simulink model "PROJETOFINALmotor"  (R2021a)
settings: Solver=VariableStepAuto  StartTime=0  StopTime=144  FixedStep=0.1  RelTol=1e-3
model workspace (MAT data in the model file):
  variavelteste = 0
libraries: autolibsharedmappedengines x2, spsACVoltageSourceLib x1, spsCurrentMeasurementLib x1, spsSeriesRLCBranchLib x1, spspowerguiLib x1
(part 2 of 4)

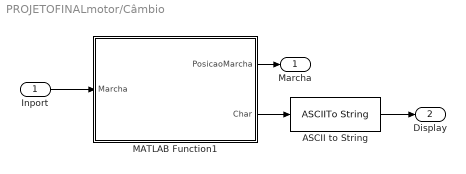
== system PROJETOFINALmotor/Câmbio ==
  Inport : Inport
  ASCII to String : ASCIIToString
  MATLAB Function1 : MATLAB Function  TreatAsAtomicUnit=on
  Marcha : Outport
  Display : Outport  Port=2
  wires:
  MATLAB Function1/1(PosicaoMarcha) -> Marcha/1
  MATLAB Function1/2(Char) -> ASCII to String/1
  ASCII to String/1 -> Display/1
  Inport/1 -> MATLAB Function1/1(Marcha)

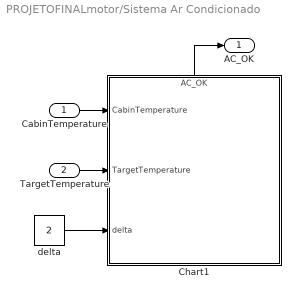
== system PROJETOFINALmotor/Sistema Ar Condicionado ==
  CabinTemperature : Inport
  TargetTemperature : Inport  Port=2
  Chart1 : Stateflow chart  TreatAsAtomicUnit=on
      settings: PortSchema="{\"entries\":[{\"content\":{\"sides\":[{\"content\":{\"connectorIds\":[\"In1\",\"In2\",\"In3\"]},\"type\":\"ConnectorPlacement.EquallySpacedRectSide\",\"uuid\":\"3dcc586e-91d0-4cd1-aed7-6dda3adf5149\"},{\"content\":{\"side\":\"RIGHT\"},\"type\":\"ConnectorPlacement.EquallySpacedRectSide\",\"uuid\":\"6a827bb4-538e-49ed-9fcc-bcf1675a0976\"},{\"content\":{\"connectorIds\":[\"Out1\"],\"side\":\"TOP\"},\"type\":\"ConnectorPlacement.EquallySpacedRectSide\",\"uuid\":\"8af03e4c-b384-4eb2-b8cc-d6be61dc8da4\"}]},\"type\":\"ConnectorPlacement.EquallySpacedConnector\",\"uuid\":\"bd7ebad6-2738-4989-9528-f935edcb496d\"}],\"packageUris\":[\"http://schema.mathworks.com/mf0/Connector/R2020b\"],\"version\":\"1.0\"}"
  delta : Constant  Value=2
  AC_OK : Outport
  wires:
  Chart1/1(AC_OK) -> AC_OK/1
  delta/1 -> Chart1/3(delta)
  CabinTemperature/1 -> Chart1/1(CabinTemperature)
  TargetTemperature/1 -> Chart1/2(TargetTemperature)

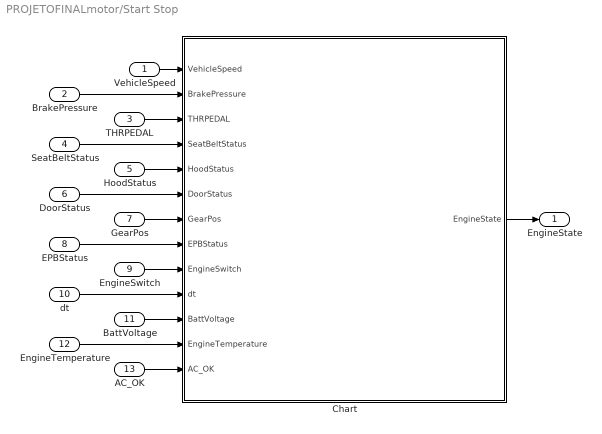
== system PROJETOFINALmotor/Start Stop ==
  VehicleSpeed : Inport
  BrakePressure : Inport  Port=2
  THRPEDAL : Inport  Port=3
  SeatBeltStatus : Inport  Port=4
  HoodStatus : Inport  Port=5
  DoorStatus : Inport  Port=6
  GearPos : Inport  Port=7
  EPBStatus : Inport  Port=8
  EngineSwitch : Inport  Port=9
  dt : Inport  Port=10
  BattVoltage : Inport  Port=11
  EngineTemperature : Inport  Port=12
  AC_OK : Inport  Port=13
  Chart : Stateflow chart  TreatAsAtomicUnit=on
  EngineState : Outport
  wires:
  Chart/1(EngineState) -> EngineState/1
  THRPEDAL/1 -> Chart/3(THRPEDAL)
  EngineTemperature/1 -> Chart/12(EngineTemperature)
  AC_OK/1 -> Chart/13(AC_OK)
  BattVoltage/1 -> Chart/11(BattVoltage)
  VehicleSpeed/1 -> Chart/1(VehicleSpeed)
  GearPos/1 -> Chart/7(GearPos)
  BrakePressure/1 -> Chart/2(BrakePressure)
  dt/1 -> Chart/10(dt)
  HoodStatus/1 -> Chart/5(HoodStatus)
  DoorStatus/1 -> Chart/6(DoorStatus)
  EngineSwitch/1 -> Chart/9(EngineSwitch)
  EPBStatus/1 -> Chart/8(EPBStatus)
  SeatBeltStatus/1 -> Chart/4(SeatBeltStatus)
